simulink subsystem "API221_ClearError"  (R2022b)
settings: Solver=VariableStepAuto  StartTime=0.0  StopTime=10.0  RelTol=1e-3
settings Model: Creator=PROSTJP  LastModifiedBy=PROSTJP

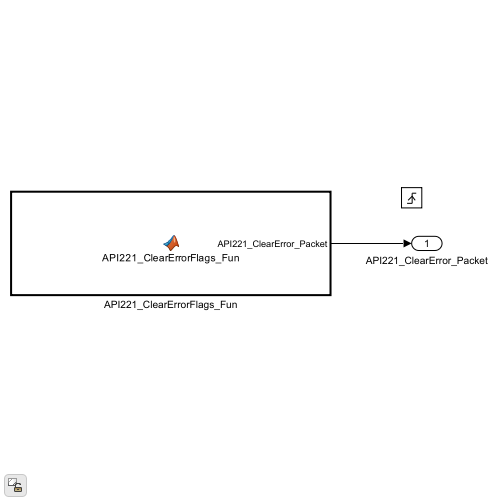
[thumbnail: Simulink's stored preview of the top-level diagram]
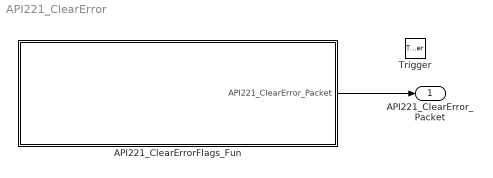
== system API221_ClearError ==
  Trigger : TriggerPort  VariantControl=(inherit)  PortDimensions=1
  API221_ClearErrorFlags_Fun : MATLAB Function  TreatAsAtomicUnit=on
  API221_ClearError_Packet : Outport
  wires:
  API221_ClearErrorFlags_Fun/1(API221_ClearError_Packet) -> API221_ClearError_Packet/1

== matlab function API221_ClearError/API221_ClearErrorFlags_Fun ==
  data: API221_ClearError_Packet output
function API221_ClearError_Packet = API221_ClearErrorFlags_Fun()
  destination = 0;
    node_id = 1;
    sdu_length = 11;
    sap = 4;
    api_id = 221;
    op_code = 2;
    cmd_fb = 0;
    frag = 0;
    mmp = 0;

    destination_source = destination + node_id * (2^4);
    opcode_compl = op_code + cmd_fb * (2^5) + frag * (2^6) + mmp * (2^7);

    motor_idx = uint8(0);
    
    header_api221 = uint8([destination_source sap sdu_length api_id opcode_compl]);
    tmp = uint8([header_api221, motor_idx]);

    API221_ClearError_Packet = zeros(100,1,'uint8');
    API221_ClearError_Packet(1:length(tmp)) = tmp;

end
